simulink model "simulink_projekt_zaliczeniowy_misk_2024_2025"  (R2023b)
settings: Solver=VariableStepAuto  StartTime=0.0  StopTime=50  MaxStep=0.1  RelTol=1e-3
settings Model: Creator=z1186362  LastModifiedBy=z1186362

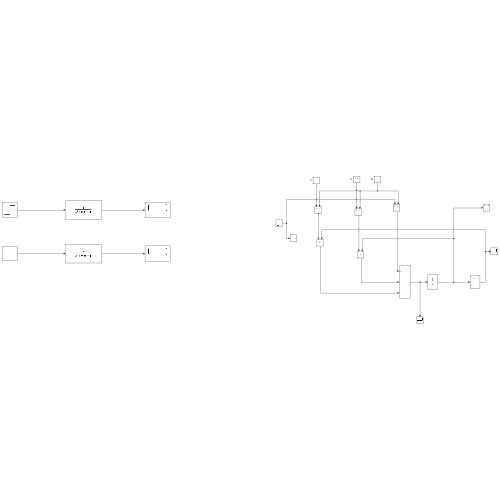
[thumbnail: Simulink's stored preview of the top-level diagram]
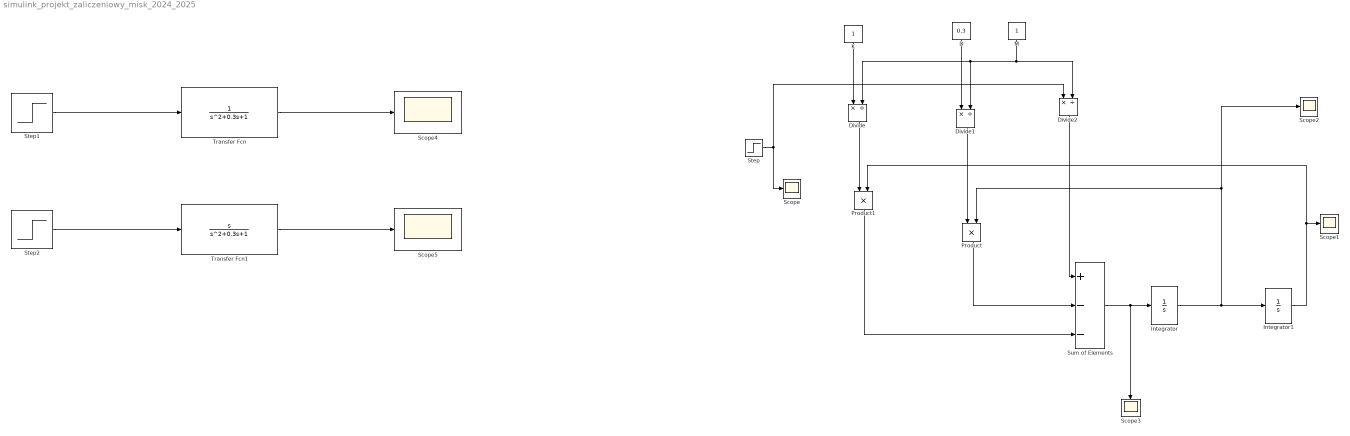
== system simulink_projekt_zaliczeniowy_misk_2024_2025 ==
  D : Constant  Value=0.3
  Divide : Product  Inputs=*/
  Divide1 : Product  Inputs=*/
  Divide2 : Product  Inputs=*/
  Integrator : Integrator
  Integrator1 : Integrator
  K : Constant
  M : Constant
  Product : Product
  Product1 : Product
  Scope{,1..5} (6 alike) : Scope
  Step : Step  Time=0  SampleTime=0
  Step1 : Step  SampleTime=0
  Step2 : Step  SampleTime=0
  Sum of Elements : Sum  Inputs=+--
  Transfer Fcn : TransferFcn  Denominator=[1 0.3 1]
  Transfer Fcn1 : TransferFcn  Numerator=[1 0]  Denominator=[1 0.3 1]
  wires:
  Step/1 -> Divide2/1, Scope/1
  K/1 -> Divide/1
  D/1 -> Divide1/1
  M/1 -> Divide2/2, Divide1/2, Divide/2
  Divide1/1 -> Product/1
  Product/1 -> Sum of Elements/2
  Divide/1 -> Product1/1
  Sum of Elements/1 -> Integrator/1, Scope3/1
  Integrator/1 -> Scope2/1, Product/2, Integrator1/1
  Integrator1/1 -> Product1/2, Scope1/1
  Divide2/1 -> Sum of Elements/1
  Product1/1 -> Sum of Elements/3
  Step1/1 -> Transfer Fcn/1
  Transfer Fcn1/1 -> Scope5/1
  Step2/1 -> Transfer Fcn1/1
  Transfer Fcn/1 -> Scope4/1
